simulink model "gm_HDLHeaderCRC_vs"  (R2024a)
settings: Solver=FixedStepDiscrete  StartTime=0.0  StopTime=stopTime  RelTol=1e-3
values from neighbouring files (symbols this model uses):
  fs = 1    [testHeaderCRC.m]
undefined symbols (not defined in the file or in its folder): clk, clk_enable, reset_x
libraries: simulink x4, dspsrcs4 x2, HDL_ieee_8021513 x2, whdlutilities x1, vivadosimlib x1
settings Model: Creator=cotti  LastModifiedBy=cotti
settings OptimizationCC: BlockReduction=off  ConditionallyExecuteInputs=off  DefaultParameterBehavior=Inlined  InheritOutputTypeSmallerThanSingle=on
settings DebuggingCC: AlgebraicLoopMsg=error  ArtificialAlgebraicLoopMsg=error  InheritedTsInSrcMsg=none  SingleTaskRateTransMsg=error  UnconnectedInputMsg=warning  UnconnectedOutputMsg=warning  UnconnectedLineMsg=warning
settings HardwareCC: ProdBitPerPointer=32  ProdBitPerSizeT=32  ProdBitPerPtrDiffT=32  ProdLargestAtomicFloat=None  ProdIntDivRoundTo=Undefined  ProdEndianess=Unspecified  ProdWordSize=32  ProdHWDeviceType=ASIC/FPGA->ASIC/FPGA  TargetBitPerLong=64  TargetBitPerPointer=64  TargetBitPerSizeT=64  TargetBitPerPtrDiffT=64  TargetLongLongMode=on  TargetIntDivRoundTo=Zero  TargetEndianess=LittleEndian  TargetWordSize=64  TargetHWDeviceType=Custom Processor->MATLAB Host Computer  ProdEqTarget=off

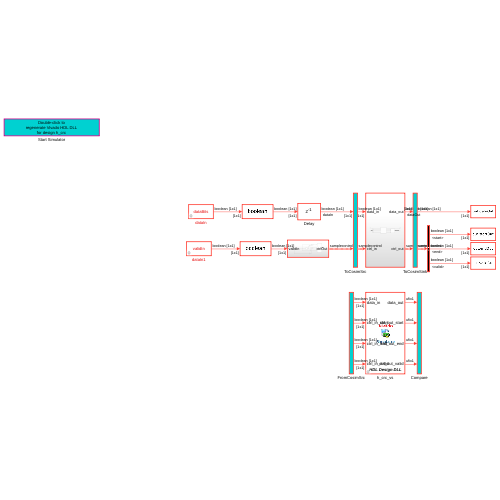
[thumbnail: Simulink's stored preview of the top-level diagram]
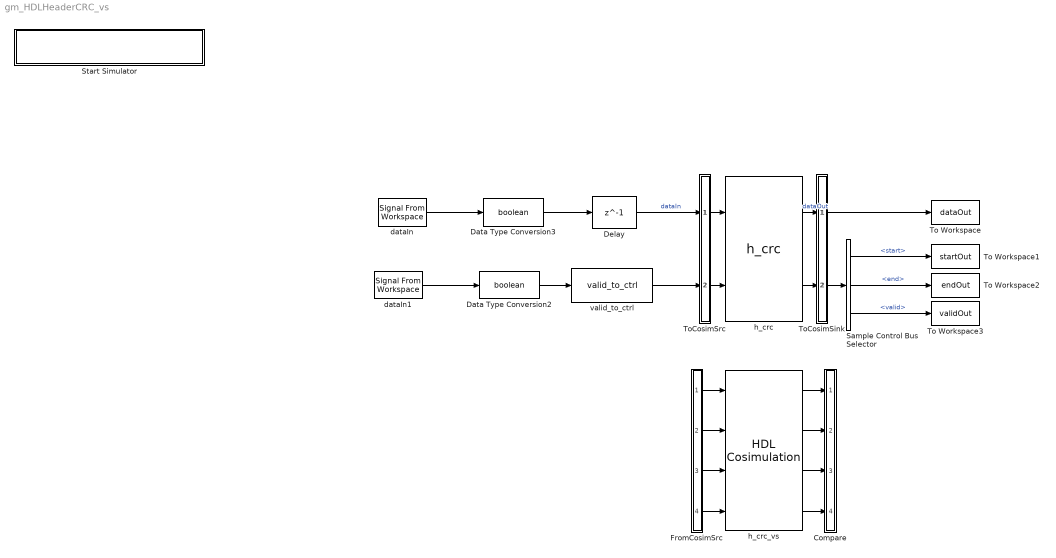
== system gm_HDLHeaderCRC_vs ==
  Compare : Subsystem
      mask Display: disp('')
  Data Type Conversion2 : DataTypeConversion  OutDataTypeStr=boolean  SaturateOnIntegerOverflow=off  RndMeth=Floor
  Data Type Conversion3 : DataTypeConversion  OutDataTypeStr=boolean  SaturateOnIntegerOverflow=off  RndMeth=Floor
  Delay : Delay  DelayLength=1  InitialCondition=0  UseCircularBuffer=on
  FromCosimSrc : Subsystem
      mask Display: disp('')
  Sample Control Bus Selector : whdlutilities/Sample Control Bus Selector  OutputSignals=start,end,valid
  Start Simulator : Subsystem
      settings: OpenFcn=|
      | cosimDirName = pwd;
      | cd 'hdl_prj/hdlsrc/HDLHeaderCRC';
      | [s,r] = system('vivado -mode batch -source gm_HDLHeaderCRC_vs.tcl','-echo');
      | cd (cosimDirName);
      | clear cosimDirName;
      | if s
      |    error('Failed to create Vivado HDL design DLL using script gm_HDLHeaderCRC_vs.tcl.');
      | end
      mask Display: disp('Double-click to\nregenerate Vivado HDL DLL\nfor design h_crc')
  To Workspace : ToWorkspace  VariableName=dataOut  SampleTime=1/fs
      settings: Save2DSignal=2-D array (concatenate along first dimension)
  To Workspace1 : ToWorkspace  VariableName=startOut  SampleTime=1/fs
      settings: Save2DSignal=2-D array (concatenate along first dimension)
  To Workspace2 : ToWorkspace  VariableName=endOut  SampleTime=1/fs
      settings: Save2DSignal=2-D array (concatenate along first dimension)
  To Workspace3 : ToWorkspace  VariableName=validOut  SampleTime=1/fs
      settings: Save2DSignal=2-D array (concatenate along first dimension)
  ToCosimSink : Subsystem
      mask Display: disp('')
  ToCosimSrc : Subsystem
      mask Display: disp('')
  dataIn : dspsrcs4/Signal From Workspace  X=dataBits  Ts=1/fs  nsamps=1  OutputAfterFinalValue=Setting to zero  ignoreOrWarnInputAndFrameLengths=off  OutputFrames=off
  dataIn1 : dspsrcs4/Signal From Workspace  X=validIn  Ts=1/fs  nsamps=1  OutputAfterFinalValue=Setting to zero  ignoreOrWarnInputAndFrameLengths=off  OutputFrames=off
  h_crc : HDL_ieee_8021513/h_crc  SystemSampleTime=-1  VariantActivationTime=update diagram  AllowFlexibleInterface=on  Latency=0  AutoFrameSizeCalculation=off
      settings: SourceProductName=HDL IEEE 8021513
  h_crc_vs : vivadosimlib/HDL Cosimulation  PortPaths=/h_crc/data_in;/h_crc/ctrl_in_start;/h_crc/ctrl_in_end;/h_crc/ctrl_in_valid;/h_crc/data_out;/h_crc/ctrl_out_start;/h_crc/ctrl_out_end;/h_crc/ctrl_out_valid  PortModes=[1 1 1 1 2 2 2 2 ]  PortTimes=[-1 -1 -1 -1 1 1 1 1 ]  PortSigns=[-1 -1 -1 -1 0 0 0 0 ]  PortFracLengths=[0,0,0,0,0,0,0,0]  PortWordLengths=[-1,-1,-1,-1,1,1,1,1]  PortHDLWordSizes=[1,1,1,1,1,1,1,1]  CommLocal=on  CommSharedMemory=on  CommPortNumber=4449  CommShowInfo=on  ClockPaths=clk;clk_enable;reset_x;  ClockModes=[2 4 3]  ClockTimes=[1e-08 3.7e-08 2.7e-08]  TclPostSimCommand="puts \"done\""  TimingMode=ns  TimingScaleFactor=10  idxCellArray={'UNUSED_VAR'}  CosimBypass=Full Simulation  AllowDirectFeedthrough=on  ProductName=EDA Simulator Link VS  RunAutoTimescale=off  HdlClocks=0  PreRunTime=40  PreRunTimeUnit=ns
  valid_to_ctrl : HDL_ieee_8021513/valid_to_ctrl  SystemSampleTime=-1  VariantActivationTime=update diagram  AllowFlexibleInterface=on  Latency=0  AutoFrameSizeCalculation=off
      settings: SourceProductName=HDL IEEE 8021513
  wires:
  Sample Control Bus Selector/2 -> To Workspace2/1  "<end>"
  Sample Control Bus Selector/3 -> To Workspace3/1  "<valid>"
  Sample Control Bus Selector/1 -> To Workspace1/1  "<start>"
  dataIn1/1 -> Data Type Conversion2/1
  Data Type Conversion3/1 -> Delay/1
  Data Type Conversion2/1 -> valid_to_ctrl/1
  dataIn/1 -> Data Type Conversion3/1
  ToCosimSrc/1(out1) -> h_crc/1
  ToCosimSrc/2(out2) -> h_crc/2
  h_crc/1 -> ToCosimSink/1(in1)  "dataOut"
  h_crc/2 -> ToCosimSink/2(in2)
  Delay/1 -> ToCosimSrc/1(in1)  "dataIn"
  valid_to_ctrl/1 -> ToCosimSrc/2(in2)
  ToCosimSink/1(out1) -> To Workspace/1
  ToCosimSink/2(out2) -> Sample Control Bus Selector/1
  FromCosimSrc/1(out1) -> h_crc_vs/1
  FromCosimSrc/2(out2) -> h_crc_vs/2
  FromCosimSrc/3(out3) -> h_crc_vs/3
  FromCosimSrc/4(out4) -> h_crc_vs/4
  h_crc_vs/1 -> Compare/1(in1)
  h_crc_vs/2 -> Compare/2(in2)
  h_crc_vs/3 -> Compare/3(in3)
  h_crc_vs/4 -> Compare/4(in4)

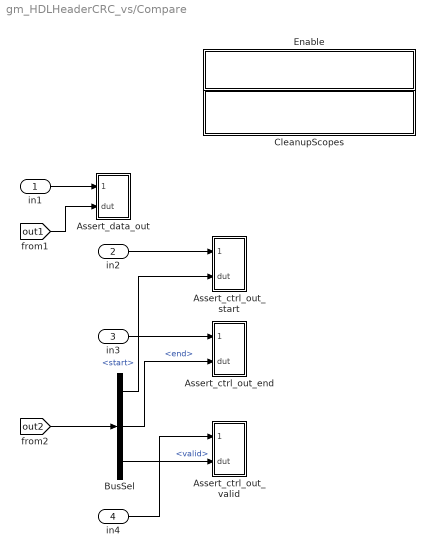
== system gm_HDLHeaderCRC_vs/Compare ==
  in1 : Inport
  in2 : Inport  Port=2
  in3 : Inport  Port=3
  in4 : Inport  Port=4
  Assert_ctrl_out_end : Subsystem
      settings: LibrarySourceBlock=hdlmdlgenlib/AssertEq
  Assert_ctrl_out_start : Subsystem
      settings: LibrarySourceBlock=hdlmdlgenlib/AssertEq
  Assert_ctrl_out_valid : Subsystem
      settings: LibrarySourceBlock=hdlmdlgenlib/AssertEq
  Assert_data_out : Subsystem
      settings: LibrarySourceBlock=hdlmdlgenlib/AssertEq
  BusSel : BusSelector  OutputSignals=start,end,valid
  CleanupScopes : Subsystem
      settings: OpenFcn=|
      | blkName = gcb; %self block
      | idx = regexp(blkName, '/CleanupScopes$', 'once');
      | blkParent = blkName(1:idx-1);
      | blks=find_system(blkParent, 'LookUnderMasks', 'all','blocktype', 'Scope');
      | for itr = 1:length(blks)
      | 	 hScopeCfg = get_param(blks{itr},'ScopeConfiguration');
      | 	 hScopeCfg.Visible = ~ hScopeCfg.Visible;
      | end
      | drawnow;
      mask Display: fprintf(message('hdlcoder:cosim:vnl_dblclick').getString());
  Enable : Subsystem
      settings: OpenFcn=|
      | blkName = gcb;
      | idx = regexp(blkName, '/Enable$', 'once');
      | blkParent = blkName(1:idx-1);
      | blks=find_system(blkParent, 'LookUnderMasks', 'all','blocktype', 'Assertion');
      | e = get_param(blks{1}, 'Enabled');
      | if strcmp(e, 'on'), f= 'off';, else, f = 'on';, end
      | for ii=1:length(blks), set_param(blks{ii}, 'Enabled', f);, end
      | set_param(gcb, 'MaskDisplay',['fprintf(message(''hdlcoder:cosim:vnl_dblclick_assertions'',','''',upper(e),'''',').getString())']);
      mask Display: fprintf(message('hdlcoder:cosim:vnl_dblclick_assertions','OFF').getString());
  wires:
  in4/1 -> Assert_ctrl_out_valid/1(cosim)
  BusSel/2 -> Assert_ctrl_out_end/2(dut)  "<end>"
  BusSel/1 -> Assert_ctrl_out_start/2(dut)  "<start>"
  in3/1 -> Assert_ctrl_out_end/1(cosim)
  in2/1 -> Assert_ctrl_out_start/1(cosim)
  BusSel/3 -> Assert_ctrl_out_valid/2(dut)  "<valid>"
  [out2] -> BusSel/1
  [out1] -> Assert_data_out/2(dut)
  in1/1 -> Assert_data_out/1(cosim)

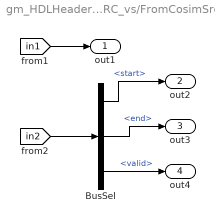
== system gm_HDLHeaderCRC_vs/FromCosimSrc ==
  BusSel : BusSelector  OutputSignals=start,end,valid
  out1 : Outport
  out2 : Outport  Port=2
  out3 : Outport  Port=3
  out4 : Outport  Port=4
  wires:
  BusSel/2 -> out3/1  "<end>"
  BusSel/1 -> out2/1  "<start>"
  BusSel/3 -> out4/1  "<valid>"
  [in2] -> BusSel/1
  [in1] -> out1/1

== system gm_HDLHeaderCRC_vs/Start Simulator ==

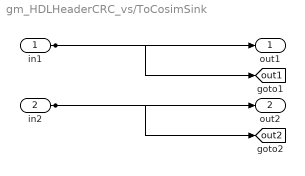
== system gm_HDLHeaderCRC_vs/ToCosimSink ==
  in1 : Inport
  in2 : Inport  Port=2
  out1 : Outport
  out2 : Outport  Port=2
  tag scope: out1=global, out2=global
  wires:
  in1/1 -> out1/1, [out1]
  in2/1 -> out2/1, [out2]

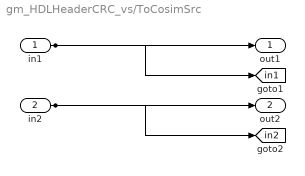
== system gm_HDLHeaderCRC_vs/ToCosimSrc ==
  in1 : Inport
  in2 : Inport  Port=2
  out1 : Outport
  out2 : Outport  Port=2
  tag scope: in1=global, in2=global
  wires:
  in1/1 -> out1/1, [in1]
  in2/1 -> out2/1, [in2]

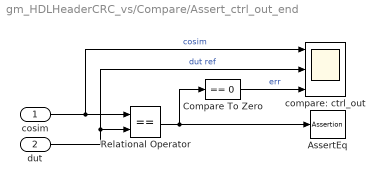
== system gm_HDLHeaderCRC_vs/Compare/Assert_ctrl_out_end ==
  cosim : Inport
  dut : Inport  Port=2
  AssertEq : Assertion
  Compare To Zero : simulink/Logic and Bit Operations/Compare To Zero  relop===  OutDataTypeStr=boolean
  Relational Operator : RelationalOperator  Operator===  OutDataTypeStr=boolean  InputSameDT=off
  compare: ctrl_out : Scope  NumInputPorts=3
  wires:
  Compare To Zero/1 -> compare: ctrl_out/3  "err"
  Relational Operator/1 -> Compare To Zero/1, AssertEq/1
  cosim/1 -> compare: ctrl_out/1, Relational Operator/1  "cosim"
  dut/1 -> compare: ctrl_out/2, Relational Operator/2  "dut ref"

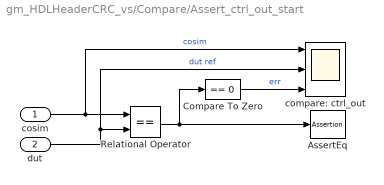
== system gm_HDLHeaderCRC_vs/Compare/Assert_ctrl_out_start ==
  cosim : Inport
  dut : Inport  Port=2
  AssertEq : Assertion
  Compare To Zero : simulink/Logic and Bit Operations/Compare To Zero  relop===  OutDataTypeStr=boolean
  Relational Operator : RelationalOperator  Operator===  OutDataTypeStr=boolean  InputSameDT=off
  compare: ctrl_out : Scope  NumInputPorts=3
  wires:
  Compare To Zero/1 -> compare: ctrl_out/3  "err"
  Relational Operator/1 -> Compare To Zero/1, AssertEq/1
  cosim/1 -> compare: ctrl_out/1, Relational Operator/1  "cosim"
  dut/1 -> compare: ctrl_out/2, Relational Operator/2  "dut ref"

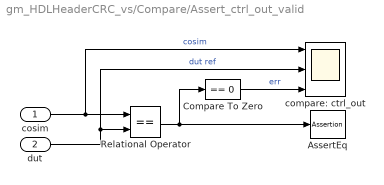
== system gm_HDLHeaderCRC_vs/Compare/Assert_ctrl_out_valid ==
  cosim : Inport
  dut : Inport  Port=2
  AssertEq : Assertion
  Compare To Zero : simulink/Logic and Bit Operations/Compare To Zero  relop===  OutDataTypeStr=boolean
  Relational Operator : RelationalOperator  Operator===  OutDataTypeStr=boolean  InputSameDT=off
  compare: ctrl_out : Scope  NumInputPorts=3
  wires:
  Compare To Zero/1 -> compare: ctrl_out/3  "err"
  Relational Operator/1 -> Compare To Zero/1, AssertEq/1
  cosim/1 -> compare: ctrl_out/1, Relational Operator/1  "cosim"
  dut/1 -> compare: ctrl_out/2, Relational Operator/2  "dut ref"

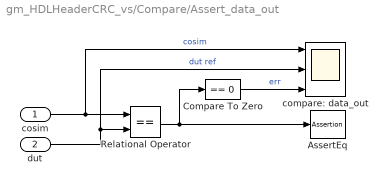
== system gm_HDLHeaderCRC_vs/Compare/Assert_data_out ==
  cosim : Inport
  dut : Inport  Port=2
  AssertEq : Assertion
  Compare To Zero : simulink/Logic and Bit Operations/Compare To Zero  relop===  OutDataTypeStr=boolean
  Relational Operator : RelationalOperator  Operator===  OutDataTypeStr=boolean  InputSameDT=off
  compare: data_out : Scope  NumInputPorts=3
  wires:
  Compare To Zero/1 -> compare: data_out/3  "err"
  Relational Operator/1 -> Compare To Zero/1, AssertEq/1
  cosim/1 -> compare: data_out/1, Relational Operator/1  "cosim"
  dut/1 -> compare: data_out/2, Relational Operator/2  "dut ref"

== system gm_HDLHeaderCRC_vs/Compare/CleanupScopes ==

== system gm_HDLHeaderCRC_vs/Compare/Enable ==
